simulink model "pendulumtest_simulink"  (R2015a)
settings: Solver=ode4  StartTime=0.0  StopTime=10  FixedStep=Ts  MaxStep=Ts  RelTol=1e-8  AbsTol=1e-8
values from neighbouring files (symbols this model uses):
  Ts = 0.001    [bodediagram_0.m]    (also in bodediagram_1.m = 0.0005)
libraries: simulink x1
settings Model: Creator=jwcjdenissen  LastModifiedBy=jwcjdenissen

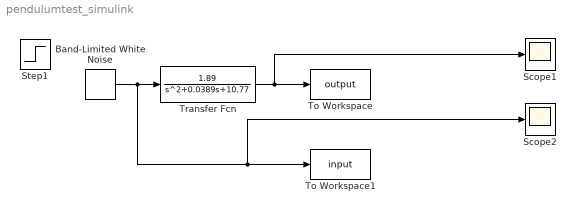
== system pendulumtest_simulink ==
  Band-Limited White Noise : simulink/Sources/Band-Limited White Noise  Cov=[0.01]  Ts=Ts  seed=[round(rand*10000)]
  Scope1 : Scope
      settings: YMin=-6  YMax=7
  Scope2 : Scope
      settings: YMin=-2000  YMax=2000
  Step1 : Step  SampleTime=0
  To Workspace : ToWorkspace  VariableName=output  SaveFormat=Timeseries  SampleTime=-1
  To Workspace1 : ToWorkspace  VariableName=input  SaveFormat=Timeseries  SampleTime=-1
  Transfer Fcn : TransferFcn  Numerator=[1.89]  Denominator=[1 0.0389 10.77]
  wires:
  Transfer Fcn/1 -> Scope1/1, To Workspace/1
  Band-Limited White Noise/1 -> Scope2/1, To Workspace1/1, Transfer Fcn/1
